simulink model "SistCompletoLazosDeCorriente_export"  (R2023b)
settings: Solver=VariableStepAuto  StartTime=0.0  StopTime=2.5  RelTol=1e-3
undefined symbols (not defined in the file): alpha_cu, b_eq, C_ts, g, J_eq, k_l, L_d, L_ls, L_q, lambda_m, magnitude, P_p, r, R_0, R_d, R_q, R_sREF, R_ts_amb, T_amb, T_sREF
settings Model: Creator=tomas  LastModifiedBy=tomas

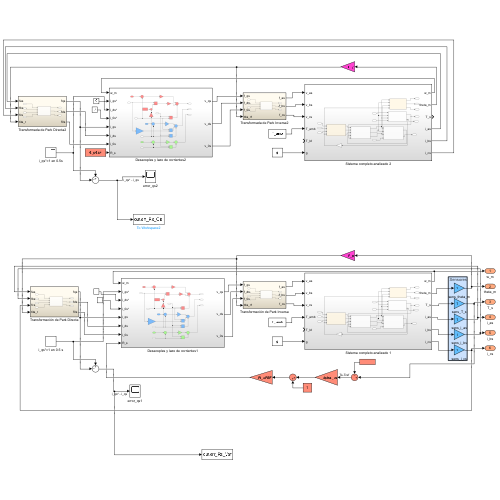
[thumbnail: Simulink's stored preview of the top-level diagram]
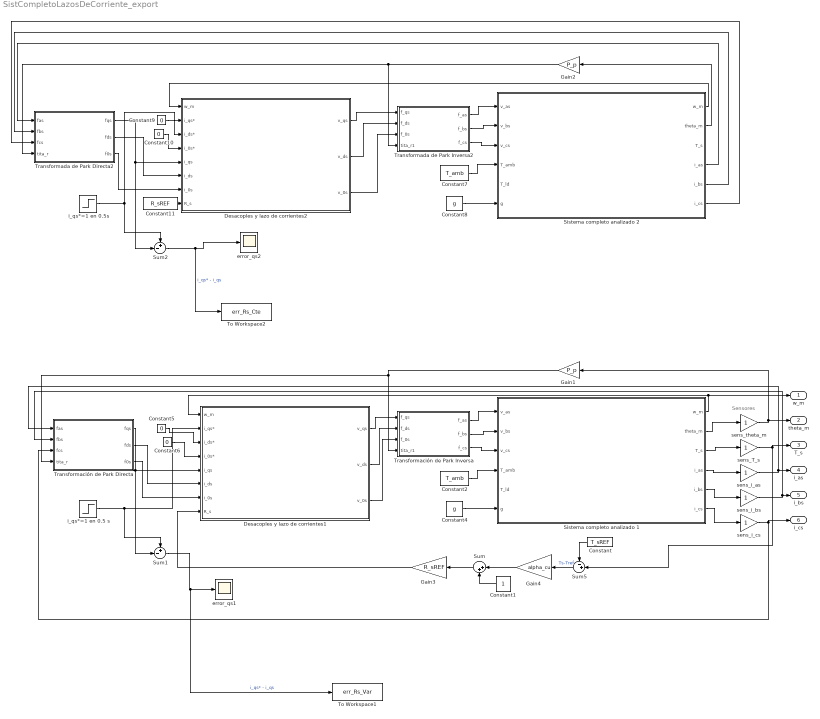
== system SistCompletoLazosDeCorriente_export ==
  note: Sensores
  Constant : Constant  Value=T_sREF
  Constant1 : Constant
  Constant{5..6,9..10} (4 alike) : Constant  Value=0
  Constant11 : Constant  Value=R_sREF
  Constant2 : Constant  Value=T_amb
  Constant4 : Constant  Value=g
  Constant7 : Constant  Value=T_amb
  Constant8 : Constant  Value=g
  Desacoples y lazo de corrientes1 : Subsystem
  Desacoples y lazo de corrientes2 : Subsystem
  Gain1 : Gain  Gain=P_p
  Gain2 : Gain  Gain=P_p
  Gain3 : Gain  Gain=R_sREF
  Gain4 : Gain  Gain=alpha_cu
  Sistema completo analizado 1 : Subsystem
  Sistema completo analizado 2 : Subsystem
  Sum : Sum  Inputs=|++
  Sum1 : Sum  Inputs=+-|
  Sum2 : Sum  Inputs=+-|
  Sum5 : Sum  Inputs=-+|
  To Workspace1 : ToWorkspace  VariableName=err_Rs_Var  SaveFormat=Structure With Time  SampleTime=-1
  To Workspace2 : ToWorkspace  VariableName=err_Rs_Cte  SaveFormat=Structure With Time  SampleTime=-1
  Transformación de Park Directa : Subsystem
  Transformación de Park Inversa : Subsystem
  Transformada de Park Directa2 : Subsystem
  Transformada de Park Inversa2 : Subsystem
  error_qs1 : Scope
  error_qs2 : Scope
  i_qs*=1 en 0.5 s : Step  Time=0.5  SampleTime=0
  i_qs*=1 en 0.5s : Step  Time=0.5  SampleTime=0
  sens_T_s : Gain
  sens_i_as : Gain
  sens_i_bs : Gain
  sens_i_cs : Gain
  sens_theta_m : Gain
  w_m : Outport
  theta_m : Outport  Port=2
  T_s : Outport  Port=3
  i_as : Outport  Port=4
  i_bs : Outport  Port=5
  i_cs : Outport  Port=6
  wires:
  Transformación de Park Inversa/2(f_bs) -> Sistema completo analizado 1/2(v_bs)
  i_qs*=1 en 0.5 s/1 -> Desacoples y lazo de corrientes1/2(i_qs*), Sum1/1
  Desacoples y lazo de corrientes1/2(v_ds) -> Transformación de Park Inversa/2(f_ds)
  Desacoples y lazo de corrientes1/1(v_qs) -> Transformación de Park Inversa/1(f_qs)
  Desacoples y lazo de corrientes1/3(v_0s) -> Transformación de Park Inversa/3(f_0s)
  Transformación de Park Directa/1(fqs) -> Desacoples y lazo de corrientes1/5(i_qs), Sum1/2
  Gain1/1 -> Transformación de Park Directa/4(tita_r), Transformación de Park Inversa/4(tita_r1)
  Transformación de Park Inversa/1(f_as) -> Sistema completo analizado 1/1(v_as)
  Sum1/1 -> To Workspace1/1, error_qs1/1  "i_qs* - i_qs"
  Transformación de Park Inversa/3(f_cs) -> Sistema completo analizado 1/3(v_cs)
  Constant2/1 -> Sistema completo analizado 1/4(T_amb)
  Transformación de Park Directa/2(fds) -> Desacoples y lazo de corrientes1/6(i_ds)
  Transformación de Park Directa/3(f0s) -> Desacoples y lazo de corrientes1/7(i_0s)
  Constant6/1 -> Desacoples y lazo de corrientes1/4(i_0s*)
  Constant5/1 -> Desacoples y lazo de corrientes1/3(i_ds*)
  Constant9/1 -> Desacoples y lazo de corrientes2/3(i_ds*)
  Desacoples y lazo de corrientes2/2(v_ds) -> Transformada de Park Inversa2/2(f_ds)
  Desacoples y lazo de corrientes2/1(v_qs) -> Transformada de Park Inversa2/1(f_qs)
  Constant10/1 -> Desacoples y lazo de corrientes2/4(i_0s*)
  Transformada de Park Directa2/3(f0s) -> Desacoples y lazo de corrientes2/7(i_0s)
  Transformada de Park Inversa2/2(f_bs) -> Sistema completo analizado 2/2(v_bs)
  i_qs*=1 en 0.5s/1 -> Desacoples y lazo de corrientes2/2(i_qs*), Sum2/1
  Sistema completo analizado 2/2(theta_m) -> Gain2/1
  Sum2/1 -> To Workspace2/1, error_qs2/1  "i_qs* - i_qs"
  Transformada de Park Directa2/2(fds) -> Desacoples y lazo de corrientes2/6(i_ds)
  Transformada de Park Inversa2/3(f_cs) -> Sistema completo analizado 2/3(v_cs)
  Gain2/1 -> Transformada de Park Directa2/4(tita_r), Transformada de Park Inversa2/4(tita_r1)
  Sistema completo analizado 2/6(i_cs) -> Transformada de Park Directa2/3(fcs)
  Sistema completo analizado 2/5(i_bs) -> Transformada de Park Directa2/2(fbs)
  Desacoples y lazo de corrientes2/3(v_0s) -> Transformada de Park Inversa2/3(f_0s)
  Transformada de Park Inversa2/1(f_as) -> Sistema completo analizado 2/1(v_as)
  Transformada de Park Directa2/1(fqs) -> Desacoples y lazo de corrientes2/5(i_qs), Sum2/2
  Sistema completo analizado 2/4(i_as) -> Transformada de Park Directa2/1(fas)
  Sistema completo analizado 2/1(w_m) -> Desacoples y lazo de corrientes2/1(w_m)
  Constant7/1 -> Sistema completo analizado 2/4(T_amb)
  Constant11/1 -> Desacoples y lazo de corrientes2/8(R_s)
  Constant4/1 -> Sistema completo analizado 1/6(g)
  Constant8/1 -> Sistema completo analizado 2/6(g)
  Gain4/1 -> Sum/1
  Sum5/1 -> Gain4/1  "Ts-Tref"
  Sum/1 -> Gain3/1
  Constant1/1 -> Sum/2
  Constant/1 -> Sum5/1
  Gain3/1 -> Desacoples y lazo de corrientes1/8(R_s)
  Sistema completo analizado 1/2(theta_m) -> sens_theta_m/1
  Sistema completo analizado 1/6(i_cs) -> sens_i_cs/1
  sens_i_as/1 -> Transformación de Park Directa/1(fas), i_as/1
  sens_theta_m/1 -> Gain1/1, theta_m/1
  Sistema completo analizado 1/3(T_s) -> sens_T_s/1
  sens_i_bs/1 -> Transformación de Park Directa/2(fbs), i_bs/1
  Sistema completo analizado 1/4(i_as) -> sens_i_as/1
  sens_i_cs/1 -> i_cs/1, Transformación de Park Directa/3(fcs)
  sens_T_s/1 -> Sum5/2, T_s/1
  Sistema completo analizado 1/5(i_bs) -> sens_i_bs/1
  Sistema completo analizado 1/1(w_m) -> w_m/1, Desacoples y lazo de corrientes1/1(w_m)

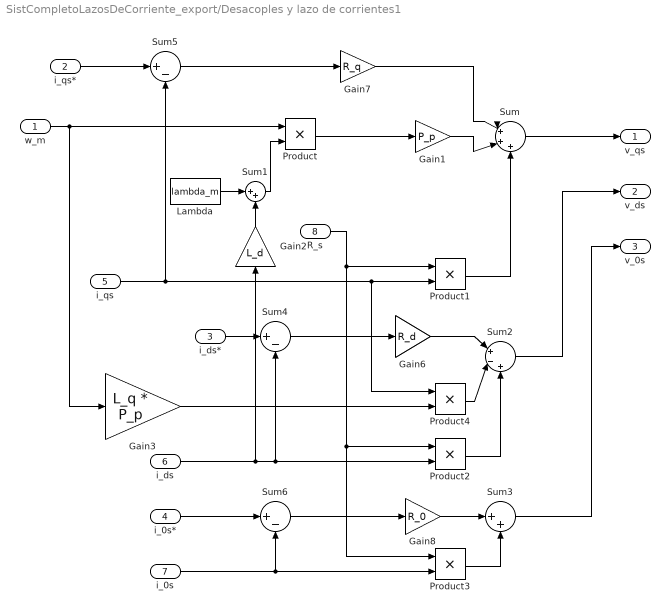
== system SistCompletoLazosDeCorriente_export/Desacoples y lazo de corrientes1 ==
  w_m : Inport
  i_qs* : Inport  Port=2
  i_ds* : Inport  Port=3
  i_0s* : Inport  Port=4
  i_qs : Inport  Port=5
  i_ds : Inport  Port=6
  i_0s : Inport  Port=7
  R_s : Inport  Port=8
  Gain1 : Gain  Gain=P_p
  Gain2 : Gain  Gain=L_d
  Gain3 : Gain  Gain=L_q * P_p
  Gain6 : Gain  Gain=R_d
  Gain7 : Gain  Gain=R_q
  Gain8 : Gain  Gain=R_0
  Lambda : Constant  Value=lambda_m
  Product{,1..4} (5 alike) : Product
  Sum : Sum  Inputs=|+++
  Sum1 : Sum  Inputs=|++
  Sum2 : Sum  Inputs=|+-+
  Sum3 : Sum  Inputs=|++
  Sum4 : Sum  Inputs=|+-
  Sum5 : Sum  Inputs=|+-
  Sum6 : Sum  Inputs=|+-
  v_qs : Outport
  v_ds : Outport  Port=2
  v_0s : Outport  Port=3
  wires:
  Sum/1 -> v_qs/1
  i_ds/1 -> Gain2/1, Product2/2, Sum4/2
  i_0s*/1 -> Sum6/1
  i_qs/1 -> Sum5/2, Product4/1, Product1/2
  Gain8/1 -> Sum3/1
  R_s/1 -> Product3/1, Product2/1, Product1/1
  i_0s/1 -> Product3/2, Sum6/2
  Sum3/1 -> v_0s/1
  Product1/1 -> Sum/3
  Gain7/1 -> Sum/1
  Sum6/1 -> Gain8/1
  Sum5/1 -> Gain7/1
  Gain6/1 -> Sum2/1
  Sum2/1 -> v_ds/1
  Gain2/1 -> Sum1/2
  Sum4/1 -> Gain6/1
  Gain3/1 -> Product4/2
  i_qs*/1 -> Sum5/1
  Product2/1 -> Sum2/3
  Gain1/1 -> Sum/2
  w_m/1 -> Gain3/1, Product/1
  Sum1/1 -> Product/2
  Lambda/1 -> Sum1/1
  Product4/1 -> Sum2/2
  Product/1 -> Gain1/1
  i_ds*/1 -> Sum4/1
  Product3/1 -> Sum3/2

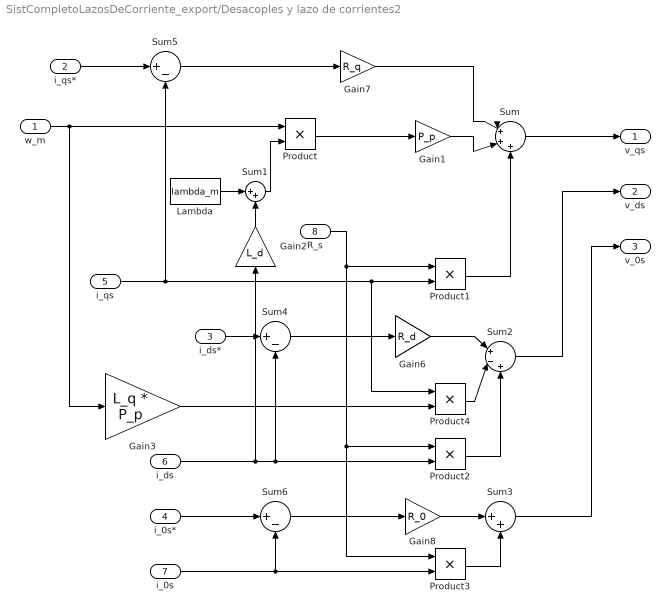
== system SistCompletoLazosDeCorriente_export/Desacoples y lazo de corrientes2 ==
  w_m : Inport
  i_qs* : Inport  Port=2
  i_ds* : Inport  Port=3
  i_0s* : Inport  Port=4
  i_qs : Inport  Port=5
  i_ds : Inport  Port=6
  i_0s : Inport  Port=7
  R_s : Inport  Port=8
  Gain1 : Gain  Gain=P_p
  Gain2 : Gain  Gain=L_d
  Gain3 : Gain  Gain=L_q * P_p
  Gain6 : Gain  Gain=R_d
  Gain7 : Gain  Gain=R_q
  Gain8 : Gain  Gain=R_0
  Lambda : Constant  Value=lambda_m
  Product{,1..4} (5 alike) : Product
  Sum : Sum  Inputs=|+++
  Sum1 : Sum  Inputs=|++
  Sum2 : Sum  Inputs=|+-+
  Sum3 : Sum  Inputs=|++
  Sum4 : Sum  Inputs=|+-
  Sum5 : Sum  Inputs=|+-
  Sum6 : Sum  Inputs=|+-
  v_qs : Outport
  v_ds : Outport  Port=2
  v_0s : Outport  Port=3
  wires:
  Sum/1 -> v_qs/1
  i_ds/1 -> Gain2/1, Product2/2, Sum4/2
  i_0s*/1 -> Sum6/1
  i_qs/1 -> Sum5/2, Product4/1, Product1/2
  Gain8/1 -> Sum3/1
  R_s/1 -> Product3/1, Product2/1, Product1/1
  i_0s/1 -> Product3/2, Sum6/2
  Sum3/1 -> v_0s/1
  Product1/1 -> Sum/3
  Gain7/1 -> Sum/1
  Sum6/1 -> Gain8/1
  Sum5/1 -> Gain7/1
  Gain6/1 -> Sum2/1
  Sum2/1 -> v_ds/1
  Gain2/1 -> Sum1/2
  Sum4/1 -> Gain6/1
  Gain3/1 -> Product4/2
  i_qs*/1 -> Sum5/1
  Product2/1 -> Sum2/3
  Gain1/1 -> Sum/2
  w_m/1 -> Gain3/1, Product/1
  Sum1/1 -> Product/2
  Lambda/1 -> Sum1/1
  Product4/1 -> Sum2/2
  Product/1 -> Gain1/1
  i_ds*/1 -> Sum4/1
  Product3/1 -> Sum3/2

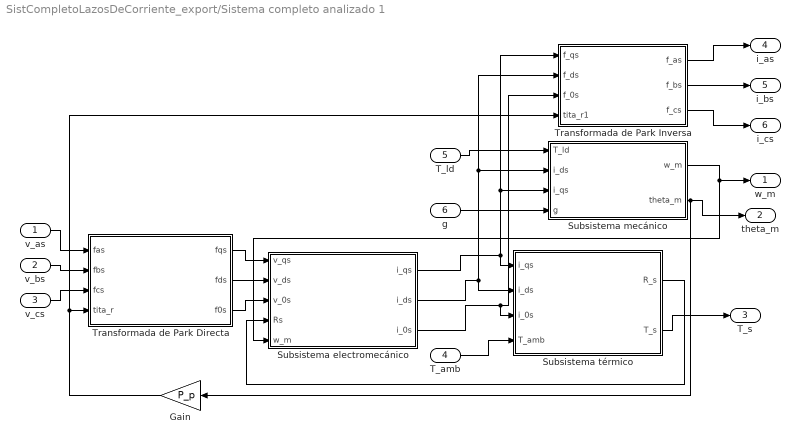
== system SistCompletoLazosDeCorriente_export/Sistema completo analizado 1 ==
  v_as : Inport
  v_bs : Inport  Port=2
  v_cs : Inport  Port=3
  T_amb : Inport  Port=4
  T_ld : Inport  Port=5
  g : Inport  Port=6
  Gain : Gain  Gain=P_p
  Subsistema electromecánico : Subsystem
  Subsistema mecánico : Subsystem
  Subsistema térmico : Subsystem
  Transformada de Park Directa : Subsystem
  Transformada de Park Inversa : Subsystem
  w_m : Outport
  theta_m : Outport  Port=2
  T_s : Outport  Port=3
  i_as : Outport  Port=4
  i_bs : Outport  Port=5
  i_cs : Outport  Port=6
  wires:
  Transformada de Park Inversa/3(f_cs) -> i_cs/1
  Subsistema mecánico/1(w_m) -> w_m/1, Subsistema electromecánico/5(w_m)
  Subsistema electromecánico/3(i_0s) -> Transformada de Park Inversa/3(f_0s), Subsistema térmico/3(i_0s)
  Transformada de Park Directa/1(fqs) -> Subsistema electromecánico/1(v_qs)
  Subsistema térmico/2(T_s) -> T_s/1
  Transformada de Park Directa/3(f0s) -> Subsistema electromecánico/3(v_0s)
  Subsistema electromecánico/2(i_ds) -> Transformada de Park Inversa/2(f_ds), Subsistema mecánico/2(i_ds), Subsistema térmico/2(i_ds)
  Gain/1 -> Transformada de Park Inversa/4(tita_r1), Transformada de Park Directa/4(tita_r)
  T_ld/1 -> Subsistema mecánico/1(T_ld)
  Transformada de Park Directa/2(fds) -> Subsistema electromecánico/2(v_ds)
  Transformada de Park Inversa/2(f_bs) -> i_bs/1
  v_bs/1 -> Transformada de Park Directa/2(fbs)
  T_amb/1 -> Subsistema térmico/4(T_amb)
  Transformada de Park Inversa/1(f_as) -> i_as/1
  v_as/1 -> Transformada de Park Directa/1(fas)
  Subsistema mecánico/2(theta_m) -> Gain/1, theta_m/1
  v_cs/1 -> Transformada de Park Directa/3(fcs)
  Subsistema electromecánico/1(i_qs) -> Subsistema térmico/1(i_qs), Subsistema mecánico/3(i_qs), Transformada de Park Inversa/1(f_qs)
  Subsistema térmico/1(R_s) -> Subsistema electromecánico/4(Rs)
  g/1 -> Subsistema mecánico/4(g)

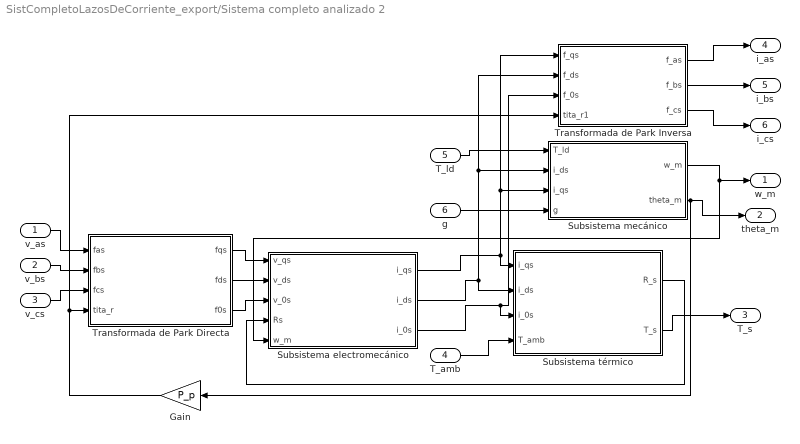
== system SistCompletoLazosDeCorriente_export/Sistema completo analizado 2 ==
  v_as : Inport
  v_bs : Inport  Port=2
  v_cs : Inport  Port=3
  T_amb : Inport  Port=4
  T_ld : Inport  Port=5
  g : Inport  Port=6
  Gain : Gain  Gain=P_p
  Subsistema electromecánico : Subsystem
  Subsistema mecánico : Subsystem
  Subsistema térmico : Subsystem
  Transformada de Park Directa : Subsystem
  Transformada de Park Inversa : Subsystem
  w_m : Outport
  theta_m : Outport  Port=2
  T_s : Outport  Port=3
  i_as : Outport  Port=4
  i_bs : Outport  Port=5
  i_cs : Outport  Port=6
  wires:
  Transformada de Park Inversa/3(f_cs) -> i_cs/1
  Subsistema mecánico/1(w_m) -> w_m/1, Subsistema electromecánico/5(w_m)
  Subsistema electromecánico/3(i_0s) -> Transformada de Park Inversa/3(f_0s), Subsistema térmico/3(i_0s)
  Transformada de Park Directa/1(fqs) -> Subsistema electromecánico/1(v_qs)
  Subsistema térmico/2(T_s) -> T_s/1
  Transformada de Park Directa/3(f0s) -> Subsistema electromecánico/3(v_0s)
  Subsistema electromecánico/2(i_ds) -> Transformada de Park Inversa/2(f_ds), Subsistema mecánico/2(i_ds), Subsistema térmico/2(i_ds)
  Gain/1 -> Transformada de Park Inversa/4(tita_r1), Transformada de Park Directa/4(tita_r)
  T_ld/1 -> Subsistema mecánico/1(T_ld)
  Transformada de Park Directa/2(fds) -> Subsistema electromecánico/2(v_ds)
  Transformada de Park Inversa/2(f_bs) -> i_bs/1
  v_bs/1 -> Transformada de Park Directa/2(fbs)
  T_amb/1 -> Subsistema térmico/4(T_amb)
  Transformada de Park Inversa/1(f_as) -> i_as/1
  v_as/1 -> Transformada de Park Directa/1(fas)
  Subsistema mecánico/2(theta_m) -> Gain/1, theta_m/1
  v_cs/1 -> Transformada de Park Directa/3(fcs)
  Subsistema electromecánico/1(i_qs) -> Subsistema térmico/1(i_qs), Subsistema mecánico/3(i_qs), Transformada de Park Inversa/1(f_qs)
  Subsistema térmico/1(R_s) -> Subsistema electromecánico/4(Rs)
  g/1 -> Subsistema mecánico/4(g)

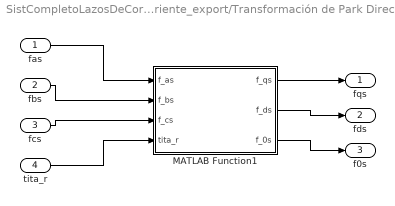
== system SistCompletoLazosDeCorriente_export/Transformación de Park Directa ==
  fas : Inport
  fbs : Inport  Port=2
  fcs : Inport  Port=3
  tita_r : Inport  Port=4
  MATLAB Function1 : MATLAB Function  TreatAsAtomicUnit=on
  fqs : Outport
  fds : Outport  Port=2
  f0s : Outport  Port=3
  wires:
  fas/1 -> MATLAB Function1/1(f_as)
  MATLAB Function1/3(f_0s) -> f0s/1
  MATLAB Function1/2(f_ds) -> fds/1
  fbs/1 -> MATLAB Function1/2(f_bs)
  fcs/1 -> MATLAB Function1/3(f_cs)
  tita_r/1 -> MATLAB Function1/4(tita_r)
  MATLAB Function1/1(f_qs) -> fqs/1

== system SistCompletoLazosDeCorriente_export/Transformación de Park Inversa ==
  f_qs : Inport
  f_ds : Inport  Port=2
  f_0s : Inport  Port=3
  tita_r1 : Inport  Port=4
  MATLAB Function2 : MATLAB Function  TreatAsAtomicUnit=on
  f_as : Outport
  f_bs : Outport  Port=2
  f_cs : Outport  Port=3
  wires:
  tita_r1/1 -> MATLAB Function2/4(tita_r)
  MATLAB Function2/2(f_bs) -> f_bs/1
  MATLAB Function2/1(f_as) -> f_as/1
  f_ds/1 -> MATLAB Function2/2(f_ds)
  MATLAB Function2/3(f_cs) -> f_cs/1
  f_0s/1 -> MATLAB Function2/3(f_0s)
  f_qs/1 -> MATLAB Function2/1(f_qs)

== system SistCompletoLazosDeCorriente_export/Transformada de Park Directa2 ==
  fas : Inport
  fbs : Inport  Port=2
  fcs : Inport  Port=3
  tita_r : Inport  Port=4
  MATLAB Function1 : MATLAB Function  TreatAsAtomicUnit=on
  fqs : Outport
  fds : Outport  Port=2
  f0s : Outport  Port=3
  wires:
  fas/1 -> MATLAB Function1/1(f_as)
  MATLAB Function1/3(f_0s) -> f0s/1
  MATLAB Function1/2(f_ds) -> fds/1
  fbs/1 -> MATLAB Function1/2(f_bs)
  fcs/1 -> MATLAB Function1/3(f_cs)
  tita_r/1 -> MATLAB Function1/4(tita_r)
  MATLAB Function1/1(f_qs) -> fqs/1

== system SistCompletoLazosDeCorriente_export/Transformada de Park Inversa2 ==
  f_qs : Inport
  f_ds : Inport  Port=2
  f_0s : Inport  Port=3
  tita_r1 : Inport  Port=4
  MATLAB Function2 : MATLAB Function  TreatAsAtomicUnit=on
  f_as : Outport
  f_bs : Outport  Port=2
  f_cs : Outport  Port=3
  wires:
  tita_r1/1 -> MATLAB Function2/4(tita_r)
  MATLAB Function2/2(f_bs) -> f_bs/1
  MATLAB Function2/1(f_as) -> f_as/1
  f_ds/1 -> MATLAB Function2/2(f_ds)
  MATLAB Function2/3(f_cs) -> f_cs/1
  f_0s/1 -> MATLAB Function2/3(f_0s)
  f_qs/1 -> MATLAB Function2/1(f_qs)

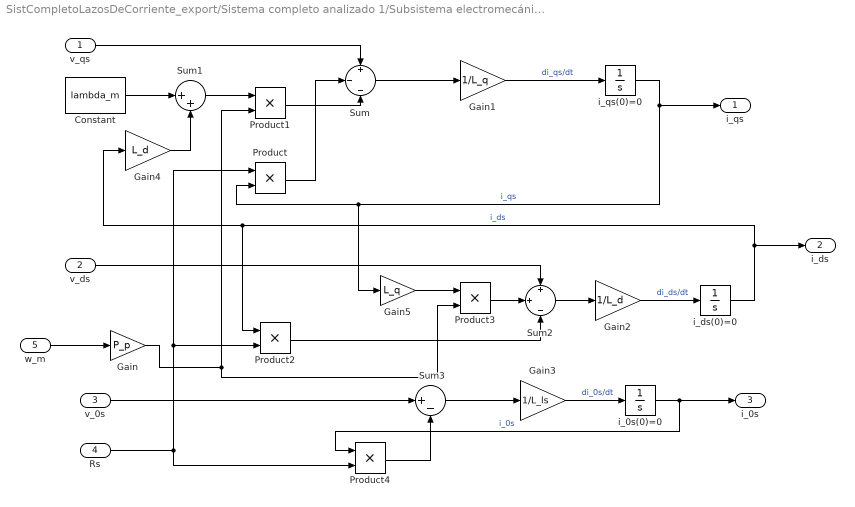
== system SistCompletoLazosDeCorriente_export/Sistema completo analizado 1/Subsistema electromecánico ==
  v_qs : Inport
  v_ds : Inport  Port=2
  v_0s : Inport  Port=3
  Rs : Inport  Port=4
  w_m : Inport  Port=5
  Constant : Constant  Value=lambda_m
  Gain : Gain  Gain=P_p
  Gain1 : Gain  Gain=1/L_q
  Gain2 : Gain  Gain=1/L_d
  Gain3 : Gain  Gain=1/L_ls
  Gain4 : Gain  Gain=L_d
  Gain5 : Gain  Gain=L_q
  Product{,1..4} (5 alike) : Product
  Sum : Sum  Inputs=+|-|-
  Sum1 : Sum  Inputs=|++
  Sum2 : Sum  Inputs=+|+|-
  Sum3 : Sum  Inputs=|+-
  i_0s(0)=0 : Integrator
  i_ds(0)=0 : Integrator
  i_qs(0)=0 : Integrator
  i_qs : Outport
  i_ds : Outport  Port=2
  i_0s : Outport  Port=3
  wires:
  Gain1/1 -> i_qs(0)=0/1  "di_qs/dt"
  Rs/1 -> Product2/2, Product/1, Product4/2
  i_qs(0)=0/1 -> Gain5/1, Product/2, i_qs/1  "i_qs"
  Sum2/1 -> Gain2/1
  Product1/1 -> Sum/3
  Product4/1 -> Sum3/2
  v_0s/1 -> Sum3/1
  Product3/1 -> Sum2/2
  Gain3/1 -> i_0s(0)=0/1  "di_0s/dt"
  Gain/1 -> Product3/2, Product1/2
  v_qs/1 -> Sum/1
  Sum1/1 -> Product1/1
  Gain5/1 -> Product3/1
  Sum3/1 -> Gain3/1
  i_0s(0)=0/1 -> Product4/1, i_0s/1  "i_0s"
  Product2/1 -> Sum2/3
  Gain2/1 -> i_ds(0)=0/1  "di_ds/dt"
  Constant/1 -> Sum1/1
  Gain4/1 -> Sum1/2
  Sum/1 -> Gain1/1
  Product/1 -> Sum/2
  w_m/1 -> Gain/1
  i_ds(0)=0/1 -> Product2/1, Gain4/1, i_ds/1  "i_ds"
  v_ds/1 -> Sum2/1

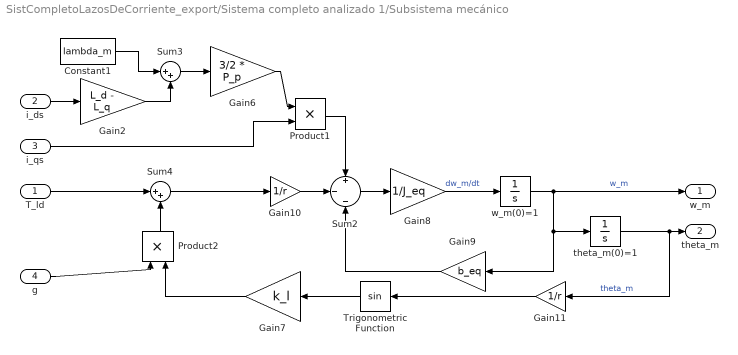
== system SistCompletoLazosDeCorriente_export/Sistema completo analizado 1/Subsistema mecánico ==
  T_ld : Inport
  i_ds : Inport  Port=2
  i_qs : Inport  Port=3
  g : Inport  Port=4
  Constant1 : Constant  Value=lambda_m
  Gain10 : Gain  Gain=1/r
  Gain11 : Gain  Gain=1/r
  Gain2 : Gain  Gain=L_d - L_q
  Gain6 : Gain  Gain=3/2 * P_p
  Gain7 : Gain  Gain=k_l
  Gain8 : Gain  Gain=1/J_eq
  Gain9 : Gain  Gain=b_eq
  Product1 : Product
  Product2 : Product
  Sum2 : Sum  Inputs=+|-|-
  Sum3 : Sum  Inputs=|++
  Sum4 : Sum  Inputs=|++
  Trigonometric Function : Trigonometry
  theta_m(0)=1 : Integrator
  w_m(0)=1 : Integrator
  w_m : Outport
  theta_m : Outport  Port=2
  wires:
  Gain7/1 -> Product2/2
  Trigonometric Function/1 -> Gain7/1
  Gain10/1 -> Sum2/2
  w_m(0)=1/1 -> w_m/1, theta_m(0)=1/1, Gain9/1  "w_m"
  Sum2/1 -> Gain8/1
  Constant1/1 -> Sum3/1
  Gain9/1 -> Sum2/3
  i_ds/1 -> Gain2/1
  Gain8/1 -> w_m(0)=1/1  "dw_m/dt"
  Product1/1 -> Sum2/1
  Gain11/1 -> Trigonometric Function/1
  T_ld/1 -> Sum4/1
  Sum4/1 -> Gain10/1
  theta_m(0)=1/1 -> Gain11/1, theta_m/1  "theta_m"
  Gain2/1 -> Sum3/2
  i_qs/1 -> Product1/2
  Sum3/1 -> Gain6/1
  g/1 -> Product2/1
  Product2/1 -> Sum4/2
  Gain6/1 -> Product1/1

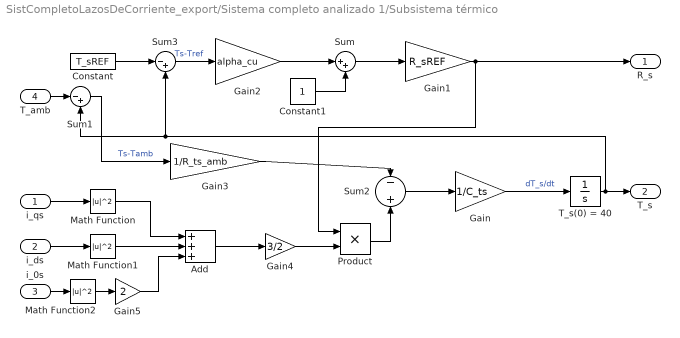
== system SistCompletoLazosDeCorriente_export/Sistema completo analizado 1/Subsistema térmico ==
  i_qs : Inport
  i_ds : Inport  Port=2
  i_0s : Inport  Port=3
  T_amb : Inport  Port=4
  Add : Sum  Inputs=+++
  Constant : Constant  Value=T_sREF
  Constant1 : Constant
  Gain : Gain  Gain=1/C_ts
  Gain1 : Gain  Gain=R_sREF
  Gain2 : Gain  Gain=alpha_cu
  Gain3 : Gain  Gain=1/R_ts_amb
  Gain4 : Gain  Gain=3/2
  Gain5 : Gain  Gain=2
  Math Function : Math  Operator=magnitude^2
  Math Function1 : Math  Operator=magnitude^2
  Math Function2 : Math  Operator=magnitude^2
  Product : Product
  Sum : Sum  Inputs=|++
  Sum1 : Sum  Inputs=|-+
  Sum2 : Sum  Inputs=-|+
  Sum3 : Sum  Inputs=|-+
  T_s(0) = 40 : Integrator  InitialCondition=40
  R_s : Outport
  T_s : Outport  Port=2
  wires:
  Gain4/1 -> Product/2
  Sum1/1 -> Gain3/1  "Ts-Tamb"
  Constant/1 -> Sum3/1
  i_ds/1 -> Math Function1/1
  Product/1 -> Sum2/2
  Math Function1/1 -> Add/2
  Gain3/1 -> Sum2/1
  i_qs/1 -> Math Function/1
  Gain5/1 -> Add/3
  Add/1 -> Gain4/1
  Gain1/1 -> Product/1, R_s/1
  Sum3/1 -> Gain2/1  "Ts-Tref"
  Math Function2/1 -> Gain5/1
  Gain2/1 -> Sum/1
  i_0s/1 -> Math Function2/1
  Math Function/1 -> Add/1
  Sum/1 -> Gain1/1
  Constant1/1 -> Sum/2
  Gain/1 -> T_s(0) = 40/1  "dT_s/dt"
  Sum2/1 -> Gain/1
  T_amb/1 -> Sum1/1
  T_s(0) = 40/1 -> T_s/1, Sum3/2, Sum1/2

== system SistCompletoLazosDeCorriente_export/Sistema completo analizado 1/Transformada de Park Directa ==
  fas : Inport
  fbs : Inport  Port=2
  fcs : Inport  Port=3
  tita_r : Inport  Port=4
  MATLAB Function1 : MATLAB Function  TreatAsAtomicUnit=on
  fqs : Outport
  fds : Outport  Port=2
  f0s : Outport  Port=3
  wires:
  fas/1 -> MATLAB Function1/1(f_as)
  MATLAB Function1/3(f_0s) -> f0s/1
  MATLAB Function1/2(f_ds) -> fds/1
  fbs/1 -> MATLAB Function1/2(f_bs)
  fcs/1 -> MATLAB Function1/3(f_cs)
  tita_r/1 -> MATLAB Function1/4(tita_r)
  MATLAB Function1/1(f_qs) -> fqs/1

== system SistCompletoLazosDeCorriente_export/Sistema completo analizado 1/Transformada de Park Inversa ==
  f_qs : Inport
  f_ds : Inport  Port=2
  f_0s : Inport  Port=3
  tita_r1 : Inport  Port=4
  MATLAB Function2 : MATLAB Function  TreatAsAtomicUnit=on
  f_as : Outport
  f_bs : Outport  Port=2
  f_cs : Outport  Port=3
  wires:
  tita_r1/1 -> MATLAB Function2/4(tita_r)
  MATLAB Function2/2(f_bs) -> f_bs/1
  MATLAB Function2/1(f_as) -> f_as/1
  f_ds/1 -> MATLAB Function2/2(f_ds)
  MATLAB Function2/3(f_cs) -> f_cs/1
  f_0s/1 -> MATLAB Function2/3(f_0s)
  f_qs/1 -> MATLAB Function2/1(f_qs)

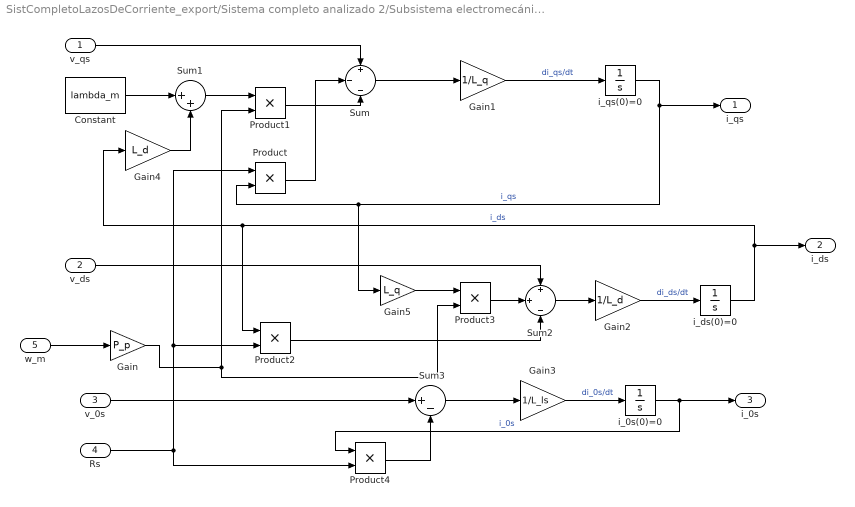
== system SistCompletoLazosDeCorriente_export/Sistema completo analizado 2/Subsistema electromecánico ==
  v_qs : Inport
  v_ds : Inport  Port=2
  v_0s : Inport  Port=3
  Rs : Inport  Port=4
  w_m : Inport  Port=5
  Constant : Constant  Value=lambda_m
  Gain : Gain  Gain=P_p
  Gain1 : Gain  Gain=1/L_q
  Gain2 : Gain  Gain=1/L_d
  Gain3 : Gain  Gain=1/L_ls
  Gain4 : Gain  Gain=L_d
  Gain5 : Gain  Gain=L_q
  Product{,1..4} (5 alike) : Product
  Sum : Sum  Inputs=+|-|-
  Sum1 : Sum  Inputs=|++
  Sum2 : Sum  Inputs=+|+|-
  Sum3 : Sum  Inputs=|+-
  i_0s(0)=0 : Integrator
  i_ds(0)=0 : Integrator
  i_qs(0)=0 : Integrator
  i_qs : Outport
  i_ds : Outport  Port=2
  i_0s : Outport  Port=3
  wires:
  Gain1/1 -> i_qs(0)=0/1  "di_qs/dt"
  Rs/1 -> Product2/2, Product/1, Product4/2
  i_qs(0)=0/1 -> Gain5/1, Product/2, i_qs/1  "i_qs"
  Sum2/1 -> Gain2/1
  Product1/1 -> Sum/3
  Product4/1 -> Sum3/2
  v_0s/1 -> Sum3/1
  Product3/1 -> Sum2/2
  Gain3/1 -> i_0s(0)=0/1  "di_0s/dt"
  Gain/1 -> Product3/2, Product1/2
  v_qs/1 -> Sum/1
  Sum1/1 -> Product1/1
  Gain5/1 -> Product3/1
  Sum3/1 -> Gain3/1
  i_0s(0)=0/1 -> Product4/1, i_0s/1  "i_0s"
  Product2/1 -> Sum2/3
  Gain2/1 -> i_ds(0)=0/1  "di_ds/dt"
  Constant/1 -> Sum1/1
  Gain4/1 -> Sum1/2
  Sum/1 -> Gain1/1
  Product/1 -> Sum/2
  w_m/1 -> Gain/1
  i_ds(0)=0/1 -> Product2/1, Gain4/1, i_ds/1  "i_ds"
  v_ds/1 -> Sum2/1

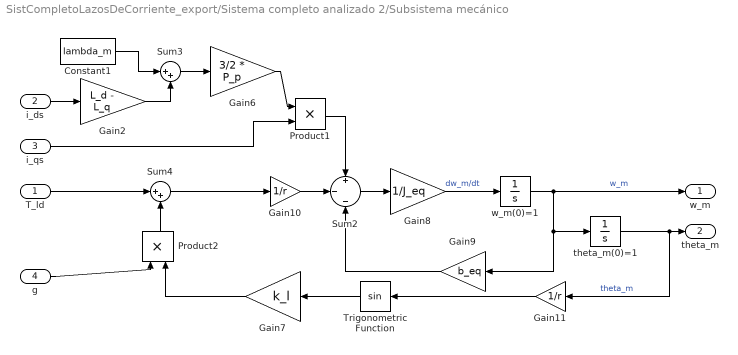
== system SistCompletoLazosDeCorriente_export/Sistema completo analizado 2/Subsistema mecánico ==
  T_ld : Inport
  i_ds : Inport  Port=2
  i_qs : Inport  Port=3
  g : Inport  Port=4
  Constant1 : Constant  Value=lambda_m
  Gain10 : Gain  Gain=1/r
  Gain11 : Gain  Gain=1/r
  Gain2 : Gain  Gain=L_d - L_q
  Gain6 : Gain  Gain=3/2 * P_p
  Gain7 : Gain  Gain=k_l
  Gain8 : Gain  Gain=1/J_eq
  Gain9 : Gain  Gain=b_eq
  Product1 : Product
  Product2 : Product
  Sum2 : Sum  Inputs=+|-|-
  Sum3 : Sum  Inputs=|++
  Sum4 : Sum  Inputs=|++
  Trigonometric Function : Trigonometry
  theta_m(0)=1 : Integrator
  w_m(0)=1 : Integrator
  w_m : Outport
  theta_m : Outport  Port=2
  wires:
  Gain7/1 -> Product2/2
  Trigonometric Function/1 -> Gain7/1
  Gain10/1 -> Sum2/2
  w_m(0)=1/1 -> w_m/1, theta_m(0)=1/1, Gain9/1  "w_m"
  Sum2/1 -> Gain8/1
  Constant1/1 -> Sum3/1
  Gain9/1 -> Sum2/3
  i_ds/1 -> Gain2/1
  Gain8/1 -> w_m(0)=1/1  "dw_m/dt"
  Product1/1 -> Sum2/1
  Gain11/1 -> Trigonometric Function/1
  T_ld/1 -> Sum4/1
  Sum4/1 -> Gain10/1
  theta_m(0)=1/1 -> Gain11/1, theta_m/1  "theta_m"
  Gain2/1 -> Sum3/2
  i_qs/1 -> Product1/2
  Sum3/1 -> Gain6/1
  g/1 -> Product2/1
  Product2/1 -> Sum4/2
  Gain6/1 -> Product1/1

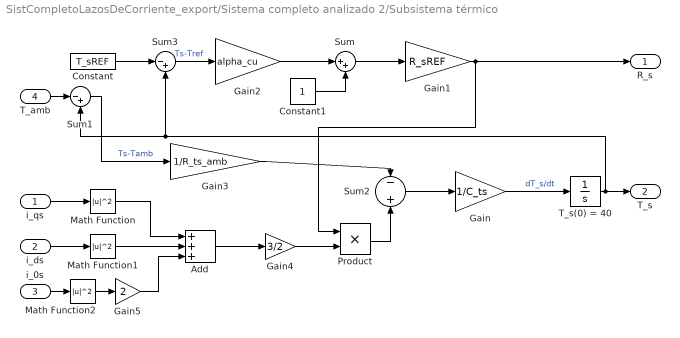
== system SistCompletoLazosDeCorriente_export/Sistema completo analizado 2/Subsistema térmico ==
  i_qs : Inport
  i_ds : Inport  Port=2
  i_0s : Inport  Port=3
  T_amb : Inport  Port=4
  Add : Sum  Inputs=+++
  Constant : Constant  Value=T_sREF
  Constant1 : Constant
  Gain : Gain  Gain=1/C_ts
  Gain1 : Gain  Gain=R_sREF
  Gain2 : Gain  Gain=alpha_cu
  Gain3 : Gain  Gain=1/R_ts_amb
  Gain4 : Gain  Gain=3/2
  Gain5 : Gain  Gain=2
  Math Function : Math  Operator=magnitude^2
  Math Function1 : Math  Operator=magnitude^2
  Math Function2 : Math  Operator=magnitude^2
  Product : Product
  Sum : Sum  Inputs=|++
  Sum1 : Sum  Inputs=|-+
  Sum2 : Sum  Inputs=-|+
  Sum3 : Sum  Inputs=|-+
  T_s(0) = 40 : Integrator  InitialCondition=40
  R_s : Outport
  T_s : Outport  Port=2
  wires:
  Gain4/1 -> Product/2
  Sum1/1 -> Gain3/1  "Ts-Tamb"
  Constant/1 -> Sum3/1
  i_ds/1 -> Math Function1/1
  Product/1 -> Sum2/2
  Math Function1/1 -> Add/2
  Gain3/1 -> Sum2/1
  i_qs/1 -> Math Function/1
  Gain5/1 -> Add/3
  Add/1 -> Gain4/1
  Gain1/1 -> Product/1, R_s/1
  Sum3/1 -> Gain2/1  "Ts-Tref"
  Math Function2/1 -> Gain5/1
  Gain2/1 -> Sum/1
  i_0s/1 -> Math Function2/1
  Math Function/1 -> Add/1
  Sum/1 -> Gain1/1
  Constant1/1 -> Sum/2
  Gain/1 -> T_s(0) = 40/1  "dT_s/dt"
  Sum2/1 -> Gain/1
  T_amb/1 -> Sum1/1
  T_s(0) = 40/1 -> T_s/1, Sum3/2, Sum1/2

== system SistCompletoLazosDeCorriente_export/Sistema completo analizado 2/Transformada de Park Directa ==
  fas : Inport
  fbs : Inport  Port=2
  fcs : Inport  Port=3
  tita_r : Inport  Port=4
  MATLAB Function1 : MATLAB Function  TreatAsAtomicUnit=on
  fqs : Outport
  fds : Outport  Port=2
  f0s : Outport  Port=3
  wires:
  fas/1 -> MATLAB Function1/1(f_as)
  MATLAB Function1/3(f_0s) -> f0s/1
  MATLAB Function1/2(f_ds) -> fds/1
  fbs/1 -> MATLAB Function1/2(f_bs)
  fcs/1 -> MATLAB Function1/3(f_cs)
  tita_r/1 -> MATLAB Function1/4(tita_r)
  MATLAB Function1/1(f_qs) -> fqs/1

== system SistCompletoLazosDeCorriente_export/Sistema completo analizado 2/Transformada de Park Inversa ==
  f_qs : Inport
  f_ds : Inport  Port=2
  f_0s : Inport  Port=3
  tita_r1 : Inport  Port=4
  MATLAB Function2 : MATLAB Function  TreatAsAtomicUnit=on
  f_as : Outport
  f_bs : Outport  Port=2
  f_cs : Outport  Port=3
  wires:
  tita_r1/1 -> MATLAB Function2/4(tita_r)
  MATLAB Function2/2(f_bs) -> f_bs/1
  MATLAB Function2/1(f_as) -> f_as/1
  f_ds/1 -> MATLAB Function2/2(f_ds)
  MATLAB Function2/3(f_cs) -> f_cs/1
  f_0s/1 -> MATLAB Function2/3(f_0s)
  f_qs/1 -> MATLAB Function2/1(f_qs)

== matlab function SistCompletoLazosDeCorriente_export/Sistema completo analizado 1/Transformada de Park Directa/MATLAB Function1 ==
  data: f_as input; f_qs output; f_bs input; f_cs input; tita_r input; f_ds output; f_0s output
function [f_qs, f_ds, f_0s] = parkDir(f_as,f_bs,f_cs,tita_r)

answer = 2/3 * [cos(tita_r), cos(tita_r - 2*pi/3), cos(tita_r + 2*pi/3);
         sin(tita_r), sin(tita_r - 2*pi/3), sin(tita_r + 2*pi/3);
         1/2, 1/2, 1/2] * [f_as;f_bs;f_cs];

f_qs = answer(1);
f_ds = answer(2);
f_0s = answer(3);

== matlab function SistCompletoLazosDeCorriente_export/Sistema completo analizado 1/Transformada de Park Inversa/MATLAB Function2 ==
  data: f_qs input; f_as output; f_ds input; f_0s input; tita_r input; f_bs output; f_cs output
function [f_as, f_bs, f_cs] = parkInv(f_qs,f_ds,f_0s,tita_r)

answer = [cos(tita_r), sin(tita_r), 1;
         cos(tita_r - 2*pi/3), sin(tita_r - 2*pi/3), 1;
         cos(tita_r + 2*pi/3), sin(tita_r + 2*pi/3), 1] * [f_qs;f_ds;f_0s]; 

f_as = answer(1);
f_bs = answer(2);
f_cs = answer(3);

== matlab function SistCompletoLazosDeCorriente_export/Transformación de Park Directa/MATLAB Function1 ==
  data: f_as input; f_qs output; f_bs input; f_cs input; tita_r input; f_ds output; f_0s output
function [f_qs, f_ds, f_0s] = parkDir(f_as,f_bs,f_cs,tita_r)

answer = 2/3 * [cos(tita_r), cos(tita_r - 2*pi/3), cos(tita_r + 2*pi/3);
         sin(tita_r), sin(tita_r - 2*pi/3), sin(tita_r + 2*pi/3);
         1/2, 1/2, 1/2] * [f_as;f_bs;f_cs];

f_qs = answer(1);
f_ds = answer(2);
f_0s = answer(3);

== matlab function SistCompletoLazosDeCorriente_export/Transformación de Park Inversa/MATLAB Function2 ==
  data: f_qs input; f_as output; f_ds input; f_0s input; tita_r input; f_bs output; f_cs output
function [f_as, f_bs, f_cs] = parkInv(f_qs,f_ds,f_0s,tita_r)

answer = [cos(tita_r), sin(tita_r), 1;
         cos(tita_r - 2*pi/3), sin(tita_r - 2*pi/3), 1;
         cos(tita_r + 2*pi/3), sin(tita_r + 2*pi/3), 1] * [f_qs;f_ds;f_0s]; 

f_as = answer(1);
f_bs = answer(2);
f_cs = answer(3);

== matlab function SistCompletoLazosDeCorriente_export/Sistema completo analizado 2/Transformada de Park Directa/MATLAB Function1 ==
  data: f_as input; f_qs output; f_bs input; f_cs input; tita_r input; f_ds output; f_0s output
function [f_qs, f_ds, f_0s] = parkDir(f_as,f_bs,f_cs,tita_r)

answer = 2/3 * [cos(tita_r), cos(tita_r - 2*pi/3), cos(tita_r + 2*pi/3);
         sin(tita_r), sin(tita_r - 2*pi/3), sin(tita_r + 2*pi/3);
         1/2, 1/2, 1/2] * [f_as;f_bs;f_cs];

f_qs = answer(1);
f_ds = answer(2);
f_0s = answer(3);

== matlab function SistCompletoLazosDeCorriente_export/Sistema completo analizado 2/Transformada de Park Inversa/MATLAB Function2 ==
  data: f_qs input; f_as output; f_ds input; f_0s input; tita_r input; f_bs output; f_cs output
function [f_as, f_bs, f_cs] = parkInv(f_qs,f_ds,f_0s,tita_r)

answer = [cos(tita_r), sin(tita_r), 1;
         cos(tita_r - 2*pi/3), sin(tita_r - 2*pi/3), 1;
         cos(tita_r + 2*pi/3), sin(tita_r + 2*pi/3), 1] * [f_qs;f_ds;f_0s]; 

f_as = answer(1);
f_bs = answer(2);
f_cs = answer(3);

== matlab function SistCompletoLazosDeCorriente_export/Transformada de Park Directa2/MATLAB Function1 ==
  data: f_as input; f_qs output; f_bs input; f_cs input; tita_r input; f_ds output; f_0s output
function [f_qs, f_ds, f_0s] = parkDir(f_as,f_bs,f_cs,tita_r)

answer = 2/3 * [cos(tita_r), cos(tita_r - 2*pi/3), cos(tita_r + 2*pi/3);
         sin(tita_r), sin(tita_r - 2*pi/3), sin(tita_r + 2*pi/3);
         1/2, 1/2, 1/2] * [f_as;f_bs;f_cs];

f_qs = answer(1);
f_ds = answer(2);
f_0s = answer(3);

== matlab function SistCompletoLazosDeCorriente_export/Transformada de Park Inversa2/MATLAB Function2 ==
  data: f_qs input; f_as output; f_ds input; f_0s input; tita_r input; f_bs output; f_cs output
function [f_as, f_bs, f_cs] = parkInv(f_qs,f_ds,f_0s,tita_r)

answer = [cos(tita_r), sin(tita_r), 1;
         cos(tita_r - 2*pi/3), sin(tita_r - 2*pi/3), 1;
         cos(tita_r + 2*pi/3), sin(tita_r + 2*pi/3), 1] * [f_qs;f_ds;f_0s]; 

f_as = answer(1);
f_bs = answer(2);
f_cs = answer(3);
